simulink model "ex1_model"  (R2021b)
settings: Solver=VariableStepAuto  StartTime=0.0  StopTime=20.0  RelTol=1e-3
settings Model: Creator=ananagirlea  LastModifiedBy=ananagirlea

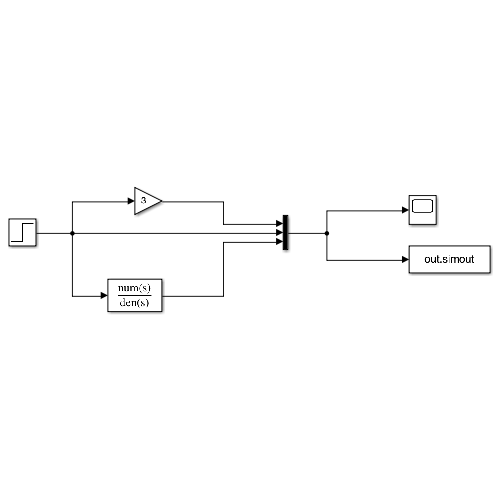
[thumbnail: Simulink's stored preview of the top-level diagram]
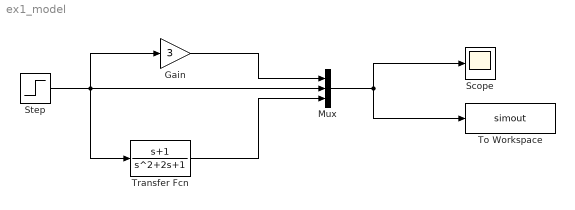
== system ex1_model ==
  Gain : Gain  Gain=3
  Mux : Mux  Inputs=3
  Scope : Scope
  Step : Step  Time=5  Before=2  After=4  SampleTime=0
  To Workspace : ToWorkspace  VariableName=simout  SaveFormat=Timeseries  SampleTime=-1
  Transfer Fcn : TransferFcn  Numerator=[1 1]
  wires:
  Transfer Fcn/1 -> Mux/3
  Step/1 -> Gain/1, Transfer Fcn/1, Mux/2
  Gain/1 -> Mux/1
  Mux/1 -> To Workspace/1, Scope/1
